simulink model "LMI_lema_5_statefeedback"  (Simulink 7.7)
settings: Solver=ode45  StartTime=0.0  StopTime=1900  RelTol=1e-3
values from neighbouring files (symbols this model uses):
  QT =     [FaseMinima.mat]    (also in FaseNaoMinima.mat; FaseNaoMinimaMudandoApenasGama.mat; settup.m = dynamics())
settings Model: Creator=Arthur  LastModifiedBy=Arthur
settings DebuggingCC: UnderspecifiedInitializationDetection=Simplified

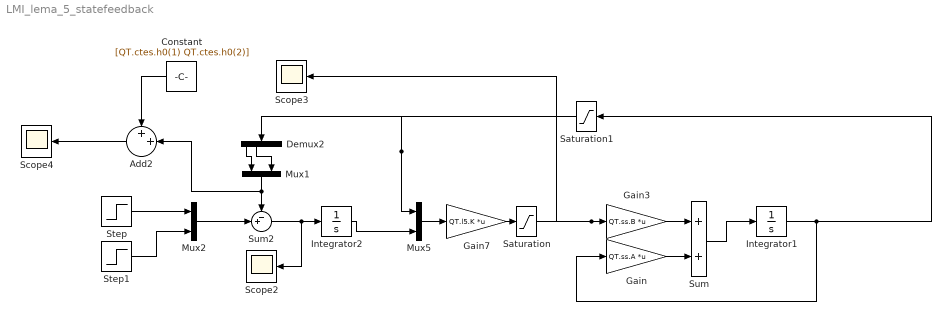
== system LMI_lema_5_statefeedback ==
  Add2 : Sum  Inputs=++|
  Constant : Constant  Value=[QT.ctes.h0(1) QT.ctes.h0(2)]
  Demux2 : Demux
  Gain : Gain  Gain=QT.ss.A  Multiplication=Matrix(K*u)
  Gain3 : Gain  Gain=QT.ss.B  Multiplication=Matrix(K*u)
  Gain7 : Gain  Gain=QT.l5.K  Multiplication=Matrix(K*u)
  Integrator1 : Integrator
  Integrator2 : Integrator
  Mux1 : Mux  Inputs=2
  Mux2 : Mux  Inputs=2
  Mux5 : Mux  Inputs=2
  Saturation : Saturate  UpperLimit=1.5  LowerLimit=-1.5
  Saturation1 : Saturate  UpperLimit=10  LowerLimit=-5
  Scope2 : Scope
      settings: YMin=-0.75  YMax=2.25  SampleTime=1
  Scope3 : Scope
      settings: YMin=-0.75  YMax=2.25  SaveName=ScopeData2  SampleInput=on  SampleTime=1
  Scope4 : Scope
      settings: TimeRange=10  SaveName=Simulado
  Step : Step  Time=300  SampleTime=0
  Step1 : Step  Time=1100  SampleTime=0
  Sum : Sum
  Sum2 : Sum  Inputs=-+|
  wires:
  Gain/1 -> Sum/2
  Gain3/1 -> Sum/1
  Step/1 -> Mux2/1
  Step1/1 -> Mux2/2
  Integrator1/1 -> Gain/1, Saturation1/1
  Sum/1 -> Integrator1/1
  Gain7/1 -> Saturation/1
  Mux5/1 -> Gain7/1
  Integrator2/1 -> Mux5/2
  Sum2/1 -> Integrator2/1, Scope2/1
  Mux2/1 -> Sum2/2
  Demux2/1 -> Mux1/1
  Demux2/2 -> Mux1/2
  Mux1/1 -> Sum2/1, Add2/2
  Saturation/1 -> Gain3/1, Scope3/1
  Saturation1/1 -> Mux5/1, Demux2/1
  Add2/1 -> Scope4/1
  Constant/1 -> Add2/1
